simulink library "VariableOrderDifferentialEquationsToolbox"  (R2020a)
settings: Solver=VariableStepAuto  StartTime=0.0  StopTime=10.0  RelTol=1e-3
(part 2 of 3)

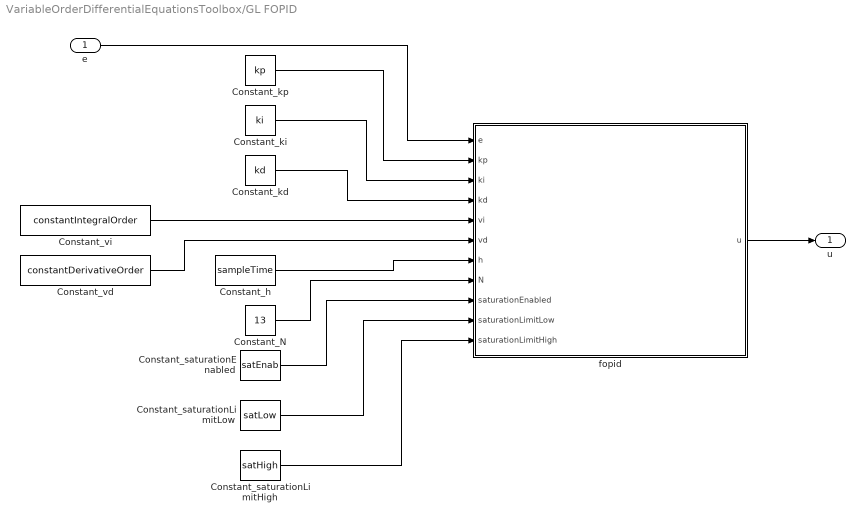
== system VariableOrderDifferentialEquationsToolbox/GL FOPID ==
  e : Inport
  Constant_N : Constant  Value=13
  Constant_h : Constant  Value=sampleTime
  Constant_kd : Constant  Value=kd
  Constant_ki : Constant  Value=ki
  Constant_kp : Constant  Value=kp
  Constant_saturationEnabled : Constant  Value=satEnab
  Constant_saturationLimitHigh : Constant  Value=satHigh
  Constant_saturationLimitLow : Constant  Value=satLow
  Constant_vd : Constant  Value=constantDerivativeOrder
  Constant_vi : Constant  Value=constantIntegralOrder
  fopid : MATLAB Function  TreatAsAtomicUnit=on  SystemSampleTime=1
  u : Outport  VectorParamsAs1DForOutWhenUnconnected=off
  wires:
  Constant_saturationLimitHigh/1 -> fopid/11(saturationLimitHigh)
  e/1 -> fopid/1(e)
  Constant_N/1 -> fopid/8(N)
  Constant_h/1 -> fopid/7(h)
  Constant_kp/1 -> fopid/2(kp)
  Constant_saturationLimitLow/1 -> fopid/10(saturationLimitLow)
  fopid/1(u) -> u/1
  Constant_saturationEnabled/1 -> fopid/9(saturationEnabled)
  Constant_kd/1 -> fopid/4(kd)
  Constant_ki/1 -> fopid/3(ki)
  Constant_vi/1 -> fopid/5(vi)
  Constant_vd/1 -> fopid/6(vd)

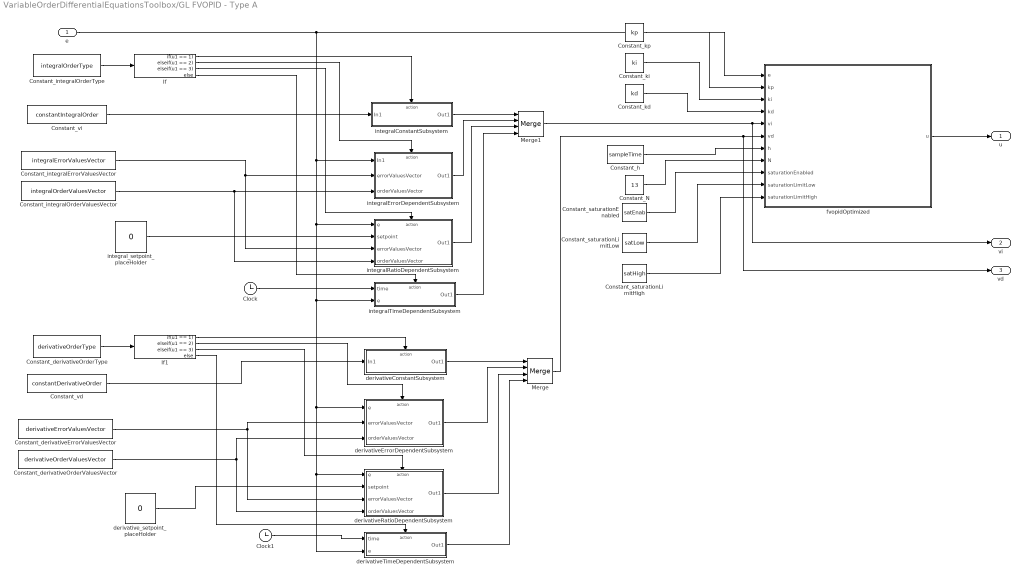
== system VariableOrderDifferentialEquationsToolbox/GL FVOPID - Type A ==
  e : Inport
  Clock : Clock
  Clock1 : Clock
  Constant_N : Constant  Value=13
  Constant_derivativeErrorValuesVector : Constant  Value=derivativeErrorValuesVector
  Constant_derivativeOrderType : Constant  Value=derivativeOrderType
  Constant_derivativeOrderValuesVector : Constant  Value=derivativeOrderValuesVector
  Constant_h : Constant  Value=sampleTime
  Constant_integralErrorValuesVector : Constant  Value=integralErrorValuesVector
  Constant_integralOrderType : Constant  Value=integralOrderType
  Constant_integralOrderValuesVector : Constant  Value=integralOrderValuesVector
  Constant_kd : Constant  Value=kd
  Constant_ki : Constant  Value=ki
  Constant_kp : Constant  Value=kp
  Constant_saturationEnabled : Constant  Value=satEnab
  Constant_saturationLimitHigh : Constant  Value=satHigh
  Constant_saturationLimitLow : Constant  Value=satLow
  Constant_vd : Constant  Value=constantDerivativeOrder
  Constant_vi : Constant  Value=constantIntegralOrder
  If : If  IfExpression=u1 == 1  ElseIfExpressions=u1 == 2, u1 == 3
  If1 : If  IfExpression=u1 == 1  ElseIfExpressions=u1 == 2, u1 == 3
  Merge : Merge  Inputs=4
  Merge1 : Merge  Inputs=4
  derivativeConstantSubsystem : Subsystem  TreatAsAtomicUnit=on
  derivativeErrorDependentSubsystem : Subsystem  TreatAsAtomicUnit=on
  derivativeRatioDependentSubsystem : Subsystem  TreatAsAtomicUnit=on
  derivativeTimeDependentSubsystem : Subsystem  TreatAsAtomicUnit=on
  derivative_setpoint_placeHolder : Constant  Value=0
  fvopidOptimized : MATLAB Function  TreatAsAtomicUnit=on  SystemSampleTime=1
  integralConstantSubsystem : Subsystem  TreatAsAtomicUnit=on
  integralErrorDependentSubsystem : Subsystem  TreatAsAtomicUnit=on
  integralRatioDependentSubsystem : Subsystem  TreatAsAtomicUnit=on
  integralTimeDependentSubsystem : Subsystem  TreatAsAtomicUnit=on
  integral_setpoint_placeHolder : Constant  Value=0
  u : Outport  VectorParamsAs1DForOutWhenUnconnected=off
  vi : Outport  Port=2  VectorParamsAs1DForOutWhenUnconnected=off
  vd : Outport  Port=3  VectorParamsAs1DForOutWhenUnconnected=off
  wires:
  Constant_saturationLimitHigh/1 -> fvopidOptimized/11(saturationLimitHigh)
  e/1 -> fvopidOptimized/1(e), integralErrorDependentSubsystem/1(In1), integralRatioDependentSubsystem/1(e), integralTimeDependentSubsystem/2(e), derivativeTimeDependentSubsystem/2(e), derivativeRatioDependentSubsystem/1(e), derivativeErrorDependentSubsystem/1(e)
  Constant_N/1 -> fvopidOptimized/8(N)
  Constant_h/1 -> fvopidOptimized/7(h)
  Constant_kp/1 -> fvopidOptimized/2(kp)
  Constant_saturationLimitLow/1 -> fvopidOptimized/10(saturationLimitLow)
  fvopidOptimized/1(u) -> u/1
  Constant_saturationEnabled/1 -> fvopidOptimized/9(saturationEnabled)
  Constant_kd/1 -> fvopidOptimized/4(kd)
  Constant_ki/1 -> fvopidOptimized/3(ki)
  Merge1/1 -> vi/1, fvopidOptimized/5(vi)
  Merge/1 -> vd/1, fvopidOptimized/6(vd)
  Constant_integralOrderType/1 -> If/1
  integralConstantSubsystem/1(Out1) -> Merge1/1
  integralErrorDependentSubsystem/1(Out1) -> Merge1/2
  Constant_vi/1 -> integralConstantSubsystem/1(In1)
  If/1 -> integralConstantSubsystem/Action
  Constant_integralErrorValuesVector/1 -> integralErrorDependentSubsystem/2(errorValuesVector), integralRatioDependentSubsystem/3(errorValuesVector)
  Constant_integralOrderValuesVector/1 -> integralRatioDependentSubsystem/4(orderValuesVector), integralErrorDependentSubsystem/3(orderValuesVector)
  integralRatioDependentSubsystem/1(Out1) -> Merge1/3
  If/2 -> integralErrorDependentSubsystem/Action
  If/4 -> integralTimeDependentSubsystem/Action
  Constant_derivativeOrderType/1 -> If1/1
  Constant_vd/1 -> derivativeConstantSubsystem/1(In1)
  derivativeConstantSubsystem/1(Out1) -> Merge/1
  If1/1 -> derivativeConstantSubsystem/Action
  If1/2 -> derivativeErrorDependentSubsystem/Action
  Constant_derivativeErrorValuesVector/1 -> derivativeErrorDependentSubsystem/2(errorValuesVector), derivativeRatioDependentSubsystem/3(errorValuesVector)
  Constant_derivativeOrderValuesVector/1 -> derivativeErrorDependentSubsystem/3(orderValuesVector), derivativeRatioDependentSubsystem/4(orderValuesVector)
  derivativeErrorDependentSubsystem/1(Out1) -> Merge/2
  derivativeRatioDependentSubsystem/1(Out1) -> Merge/3
  Clock/1 -> integralTimeDependentSubsystem/1(time)
  integralTimeDependentSubsystem/1(Out1) -> Merge1/4
  If/3 -> integralRatioDependentSubsystem/Action
  If1/3 -> derivativeRatioDependentSubsystem/Action
  If1/4 -> derivativeTimeDependentSubsystem/Action
  Clock1/1 -> derivativeTimeDependentSubsystem/1(time)
  derivativeTimeDependentSubsystem/1(Out1) -> Merge/4
  integral_setpoint_placeHolder/1 -> integralRatioDependentSubsystem/2(setpoint)
  derivative_setpoint_placeHolder/1 -> derivativeRatioDependentSubsystem/2(setpoint)

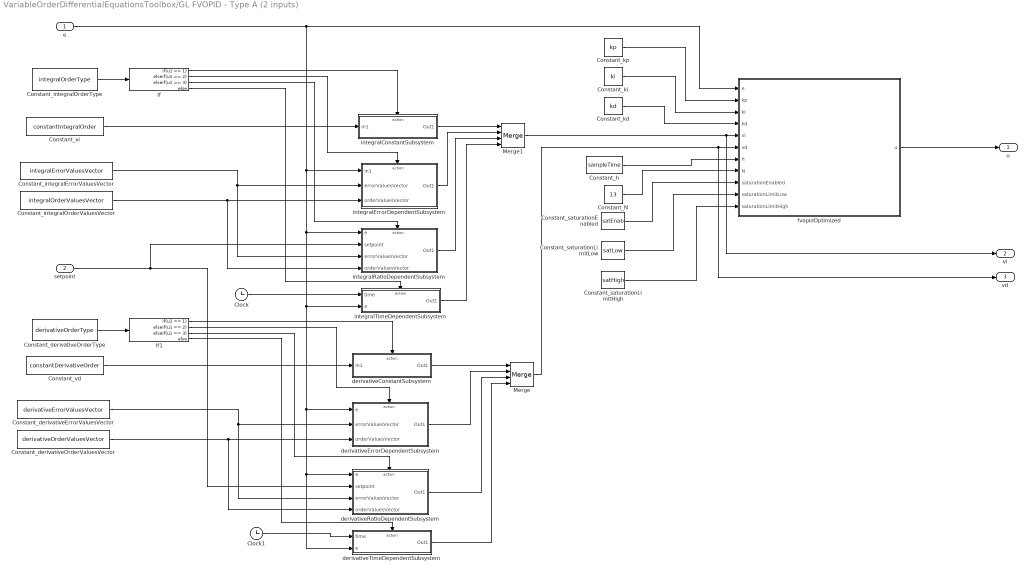
== system VariableOrderDifferentialEquationsToolbox/GL FVOPID - Type A (2 inputs) ==
  e : Inport
  setpoint : Inport  Port=2
  Clock : Clock
  Clock1 : Clock
  Constant_N : Constant  Value=13
  Constant_derivativeErrorValuesVector : Constant  Value=derivativeErrorValuesVector
  Constant_derivativeOrderType : Constant  Value=derivativeOrderType
  Constant_derivativeOrderValuesVector : Constant  Value=derivativeOrderValuesVector
  Constant_h : Constant  Value=sampleTime
  Constant_integralErrorValuesVector : Constant  Value=integralErrorValuesVector
  Constant_integralOrderType : Constant  Value=integralOrderType
  Constant_integralOrderValuesVector : Constant  Value=integralOrderValuesVector
  Constant_kd : Constant  Value=kd
  Constant_ki : Constant  Value=ki
  Constant_kp : Constant  Value=kp
  Constant_saturationEnabled : Constant  Value=satEnab
  Constant_saturationLimitHigh : Constant  Value=satHigh
  Constant_saturationLimitLow : Constant  Value=satLow
  Constant_vd : Constant  Value=constantDerivativeOrder
  Constant_vi : Constant  Value=constantIntegralOrder
  If : If  IfExpression=u1 == 1  ElseIfExpressions=u1 == 2, u1 == 3
  If1 : If  IfExpression=u1 == 1  ElseIfExpressions=u1 == 2, u1 == 3
  Merge : Merge  Inputs=4
  Merge1 : Merge  Inputs=4
  derivativeConstantSubsystem : Subsystem  TreatAsAtomicUnit=on
  derivativeErrorDependentSubsystem : Subsystem  TreatAsAtomicUnit=on
  derivativeRatioDependentSubsystem : Subsystem  TreatAsAtomicUnit=on
  derivativeTimeDependentSubsystem : Subsystem  TreatAsAtomicUnit=on
  fvopidOptimized : MATLAB Function  TreatAsAtomicUnit=on  SystemSampleTime=1
  integralConstantSubsystem : Subsystem  TreatAsAtomicUnit=on
  integralErrorDependentSubsystem : Subsystem  TreatAsAtomicUnit=on
  integralRatioDependentSubsystem : Subsystem  TreatAsAtomicUnit=on
  integralTimeDependentSubsystem : Subsystem  TreatAsAtomicUnit=on
  u : Outport  VectorParamsAs1DForOutWhenUnconnected=off
  vi : Outport  Port=2  VectorParamsAs1DForOutWhenUnconnected=off
  vd : Outport  Port=3  VectorParamsAs1DForOutWhenUnconnected=off
  wires:
  Constant_saturationLimitHigh/1 -> fvopidOptimized/11(saturationLimitHigh)
  e/1 -> integralErrorDependentSubsystem/1(In1), integralRatioDependentSubsystem/1(e), integralTimeDependentSubsystem/2(e), derivativeTimeDependentSubsystem/2(e), derivativeRatioDependentSubsystem/1(e), derivativeErrorDependentSubsystem/1(e), fvopidOptimized/1(e)
  Constant_N/1 -> fvopidOptimized/8(N)
  Constant_h/1 -> fvopidOptimized/7(h)
  Constant_kp/1 -> fvopidOptimized/2(kp)
  Constant_saturationLimitLow/1 -> fvopidOptimized/10(saturationLimitLow)
  fvopidOptimized/1(u) -> u/1
  Constant_saturationEnabled/1 -> fvopidOptimized/9(saturationEnabled)
  Constant_kd/1 -> fvopidOptimized/4(kd)
  Constant_ki/1 -> fvopidOptimized/3(ki)
  Merge1/1 -> vi/1, fvopidOptimized/5(vi)
  Merge/1 -> vd/1, fvopidOptimized/6(vd)
  Constant_integralOrderType/1 -> If/1
  integralConstantSubsystem/1(Out1) -> Merge1/1
  integralErrorDependentSubsystem/1(Out1) -> Merge1/2
  Constant_vi/1 -> integralConstantSubsystem/1(In1)
  If/1 -> integralConstantSubsystem/Action
  Constant_integralErrorValuesVector/1 -> integralErrorDependentSubsystem/2(errorValuesVector), integralRatioDependentSubsystem/3(errorValuesVector)
  Constant_integralOrderValuesVector/1 -> integralRatioDependentSubsystem/4(orderValuesVector), integralErrorDependentSubsystem/3(orderValuesVector)
  integralRatioDependentSubsystem/1(Out1) -> Merge1/3
  If/2 -> integralErrorDependentSubsystem/Action
  If/4 -> integralTimeDependentSubsystem/Action
  Constant_derivativeOrderType/1 -> If1/1
  Constant_vd/1 -> derivativeConstantSubsystem/1(In1)
  derivativeConstantSubsystem/1(Out1) -> Merge/1
  If1/1 -> derivativeConstantSubsystem/Action
  If1/2 -> derivativeErrorDependentSubsystem/Action
  Constant_derivativeErrorValuesVector/1 -> derivativeRatioDependentSubsystem/3(errorValuesVector), derivativeErrorDependentSubsystem/2(errorValuesVector)
  Constant_derivativeOrderValuesVector/1 -> derivativeRatioDependentSubsystem/4(orderValuesVector), derivativeErrorDependentSubsystem/3(orderValuesVector)
  derivativeErrorDependentSubsystem/1(Out1) -> Merge/2
  derivativeRatioDependentSubsystem/1(Out1) -> Merge/3
  Clock/1 -> integralTimeDependentSubsystem/1(time)
  integralTimeDependentSubsystem/1(Out1) -> Merge1/4
  If/3 -> integralRatioDependentSubsystem/Action
  If1/3 -> derivativeRatioDependentSubsystem/Action
  If1/4 -> derivativeTimeDependentSubsystem/Action
  Clock1/1 -> derivativeTimeDependentSubsystem/1(time)
  derivativeTimeDependentSubsystem/1(Out1) -> Merge/4
  setpoint/1 -> integralRatioDependentSubsystem/2(setpoint), derivativeRatioDependentSubsystem/2(setpoint)

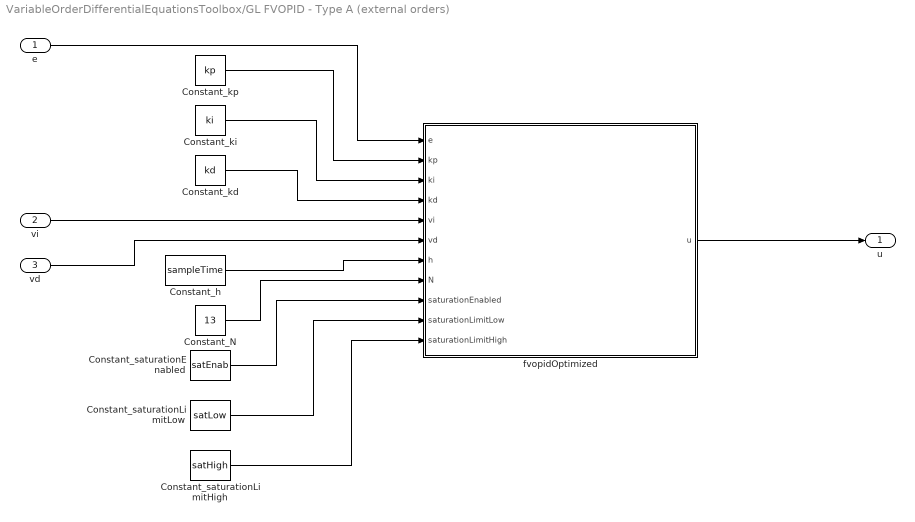
== system VariableOrderDifferentialEquationsToolbox/GL FVOPID - Type A (external orders) ==
  e : Inport
  vi : Inport  Port=2
  vd : Inport  Port=3
  Constant_N : Constant  Value=13
  Constant_h : Constant  Value=sampleTime
  Constant_kd : Constant  Value=kd
  Constant_ki : Constant  Value=ki
  Constant_kp : Constant  Value=kp
  Constant_saturationEnabled : Constant  Value=satEnab
  Constant_saturationLimitHigh : Constant  Value=satHigh
  Constant_saturationLimitLow : Constant  Value=satLow
  fvopidOptimized : MATLAB Function  TreatAsAtomicUnit=on  SystemSampleTime=1
  u : Outport  VectorParamsAs1DForOutWhenUnconnected=off
  wires:
  Constant_saturationLimitHigh/1 -> fvopidOptimized/11(saturationLimitHigh)
  e/1 -> fvopidOptimized/1(e)
  Constant_N/1 -> fvopidOptimized/8(N)
  Constant_h/1 -> fvopidOptimized/7(h)
  Constant_kp/1 -> fvopidOptimized/2(kp)
  Constant_saturationLimitLow/1 -> fvopidOptimized/10(saturationLimitLow)
  fvopidOptimized/1(u) -> u/1
  Constant_saturationEnabled/1 -> fvopidOptimized/9(saturationEnabled)
  Constant_kd/1 -> fvopidOptimized/4(kd)
  Constant_ki/1 -> fvopidOptimized/3(ki)
  vi/1 -> fvopidOptimized/5(vi)
  vd/1 -> fvopidOptimized/6(vd)

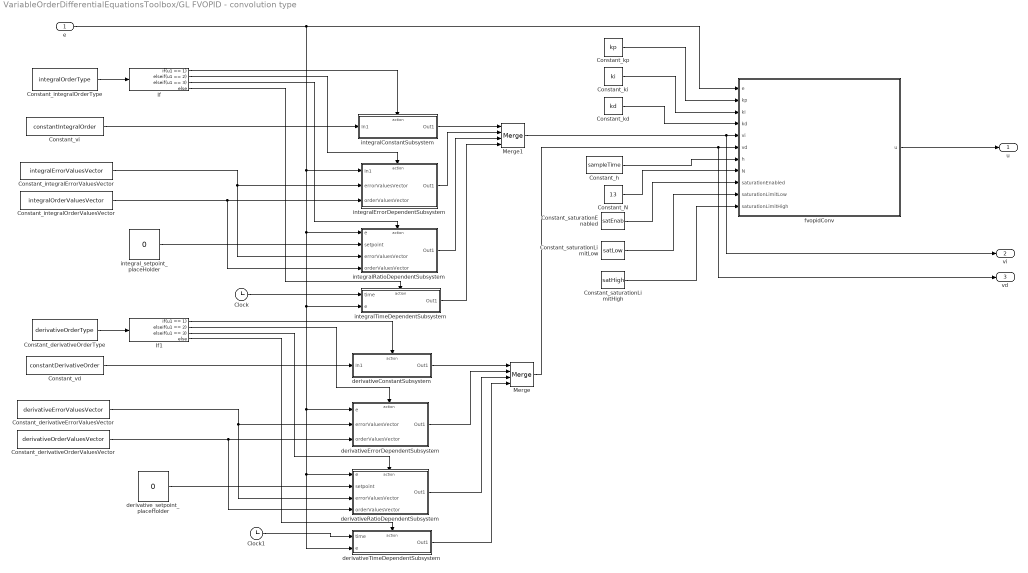
== system VariableOrderDifferentialEquationsToolbox/GL FVOPID - convolution type ==
  e : Inport
  Clock : Clock
  Clock1 : Clock
  Constant_N : Constant  Value=13
  Constant_derivativeErrorValuesVector : Constant  Value=derivativeErrorValuesVector
  Constant_derivativeOrderType : Constant  Value=derivativeOrderType
  Constant_derivativeOrderValuesVector : Constant  Value=derivativeOrderValuesVector
  Constant_h : Constant  Value=sampleTime
  Constant_integralErrorValuesVector : Constant  Value=integralErrorValuesVector
  Constant_integralOrderType : Constant  Value=integralOrderType
  Constant_integralOrderValuesVector : Constant  Value=integralOrderValuesVector
  Constant_kd : Constant  Value=kd
  Constant_ki : Constant  Value=ki
  Constant_kp : Constant  Value=kp
  Constant_saturationEnabled : Constant  Value=satEnab
  Constant_saturationLimitHigh : Constant  Value=satHigh
  Constant_saturationLimitLow : Constant  Value=satLow
  Constant_vd : Constant  Value=constantDerivativeOrder
  Constant_vi : Constant  Value=constantIntegralOrder
  If : If  IfExpression=u1 == 1  ElseIfExpressions=u1 == 2, u1 == 3
  If1 : If  IfExpression=u1 == 1  ElseIfExpressions=u1 == 2, u1 == 3
  Merge : Merge  Inputs=4
  Merge1 : Merge  Inputs=4
  derivativeConstantSubsystem : Subsystem  TreatAsAtomicUnit=on
  derivativeErrorDependentSubsystem : Subsystem  TreatAsAtomicUnit=on
  derivativeRatioDependentSubsystem : Subsystem  TreatAsAtomicUnit=on
  derivativeTimeDependentSubsystem : Subsystem  TreatAsAtomicUnit=on
  derivative_setpoint_placeHolder : Constant  Value=0
  fvopidConv : MATLAB Function  TreatAsAtomicUnit=on  SystemSampleTime=1
  integralConstantSubsystem : Subsystem  TreatAsAtomicUnit=on
  integralErrorDependentSubsystem : Subsystem  TreatAsAtomicUnit=on
  integralRatioDependentSubsystem : Subsystem  TreatAsAtomicUnit=on
  integralTimeDependentSubsystem : Subsystem  TreatAsAtomicUnit=on
  integral_setpoint_placeHolder : Constant  Value=0
  u : Outport  VectorParamsAs1DForOutWhenUnconnected=off
  vi : Outport  Port=2  VectorParamsAs1DForOutWhenUnconnected=off
  vd : Outport  Port=3  VectorParamsAs1DForOutWhenUnconnected=off
  wires:
  Constant_saturationLimitHigh/1 -> fvopidConv/11(saturationLimitHigh)
  e/1 -> integralErrorDependentSubsystem/1(In1), integralRatioDependentSubsystem/1(e), integralTimeDependentSubsystem/2(e), derivativeTimeDependentSubsystem/2(e), derivativeRatioDependentSubsystem/1(e), derivativeErrorDependentSubsystem/1(e), fvopidConv/1(e)
  Constant_N/1 -> fvopidConv/8(N)
  Constant_h/1 -> fvopidConv/7(h)
  Constant_kp/1 -> fvopidConv/2(kp)
  Constant_saturationLimitLow/1 -> fvopidConv/10(saturationLimitLow)
  fvopidConv/1(u) -> u/1
  Constant_saturationEnabled/1 -> fvopidConv/9(saturationEnabled)
  Constant_kd/1 -> fvopidConv/4(kd)
  Constant_ki/1 -> fvopidConv/3(ki)
  Merge1/1 -> vi/1, fvopidConv/5(vi)
  Merge/1 -> vd/1, fvopidConv/6(vd)
  Constant_integralOrderType/1 -> If/1
  integralConstantSubsystem/1(Out1) -> Merge1/1
  integralErrorDependentSubsystem/1(Out1) -> Merge1/2
  Constant_vi/1 -> integralConstantSubsystem/1(In1)
  If/1 -> integralConstantSubsystem/Action
  Constant_integralErrorValuesVector/1 -> integralErrorDependentSubsystem/2(errorValuesVector), integralRatioDependentSubsystem/3(errorValuesVector)
  Constant_integralOrderValuesVector/1 -> integralRatioDependentSubsystem/4(orderValuesVector), integralErrorDependentSubsystem/3(orderValuesVector)
  integralRatioDependentSubsystem/1(Out1) -> Merge1/3
  If/2 -> integralErrorDependentSubsystem/Action
  If/4 -> integralTimeDependentSubsystem/Action
  Constant_derivativeOrderType/1 -> If1/1
  Constant_vd/1 -> derivativeConstantSubsystem/1(In1)
  derivativeConstantSubsystem/1(Out1) -> Merge/1
  If1/1 -> derivativeConstantSubsystem/Action
  If1/2 -> derivativeErrorDependentSubsystem/Action
  Constant_derivativeErrorValuesVector/1 -> derivativeRatioDependentSubsystem/3(errorValuesVector), derivativeErrorDependentSubsystem/2(errorValuesVector)
  Constant_derivativeOrderValuesVector/1 -> derivativeRatioDependentSubsystem/4(orderValuesVector), derivativeErrorDependentSubsystem/3(orderValuesVector)
  derivativeErrorDependentSubsystem/1(Out1) -> Merge/2
  derivativeRatioDependentSubsystem/1(Out1) -> Merge/3
  Clock/1 -> integralTimeDependentSubsystem/1(time)
  integralTimeDependentSubsystem/1(Out1) -> Merge1/4
  If/3 -> integralRatioDependentSubsystem/Action
  If1/3 -> derivativeRatioDependentSubsystem/Action
  If1/4 -> derivativeTimeDependentSubsystem/Action
  Clock1/1 -> derivativeTimeDependentSubsystem/1(time)
  derivativeTimeDependentSubsystem/1(Out1) -> Merge/4
  integral_setpoint_placeHolder/1 -> integralRatioDependentSubsystem/2(setpoint)
  derivative_setpoint_placeHolder/1 -> derivativeRatioDependentSubsystem/2(setpoint)

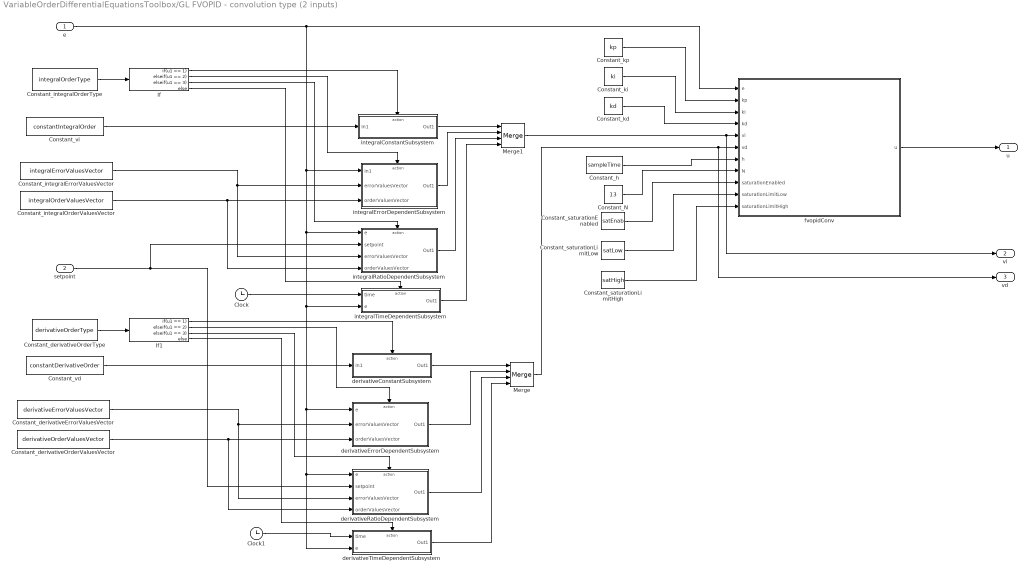
== system VariableOrderDifferentialEquationsToolbox/GL FVOPID - convolution type (2 inputs) ==
  e : Inport
  setpoint : Inport  Port=2
  Clock : Clock
  Clock1 : Clock
  Constant_N : Constant  Value=13
  Constant_derivativeErrorValuesVector : Constant  Value=derivativeErrorValuesVector
  Constant_derivativeOrderType : Constant  Value=derivativeOrderType
  Constant_derivativeOrderValuesVector : Constant  Value=derivativeOrderValuesVector
  Constant_h : Constant  Value=sampleTime
  Constant_integralErrorValuesVector : Constant  Value=integralErrorValuesVector
  Constant_integralOrderType : Constant  Value=integralOrderType
  Constant_integralOrderValuesVector : Constant  Value=integralOrderValuesVector
  Constant_kd : Constant  Value=kd
  Constant_ki : Constant  Value=ki
  Constant_kp : Constant  Value=kp
  Constant_saturationEnabled : Constant  Value=satEnab
  Constant_saturationLimitHigh : Constant  Value=satHigh
  Constant_saturationLimitLow : Constant  Value=satLow
  Constant_vd : Constant  Value=constantDerivativeOrder
  Constant_vi : Constant  Value=constantIntegralOrder
  If : If  IfExpression=u1 == 1  ElseIfExpressions=u1 == 2, u1 == 3
  If1 : If  IfExpression=u1 == 1  ElseIfExpressions=u1 == 2, u1 == 3
  Merge : Merge  Inputs=4
  Merge1 : Merge  Inputs=4
  derivativeConstantSubsystem : Subsystem  TreatAsAtomicUnit=on
  derivativeErrorDependentSubsystem : Subsystem  TreatAsAtomicUnit=on
  derivativeRatioDependentSubsystem : Subsystem  TreatAsAtomicUnit=on
  derivativeTimeDependentSubsystem : Subsystem  TreatAsAtomicUnit=on
  fvopidConv : MATLAB Function  TreatAsAtomicUnit=on  SystemSampleTime=1
  integralConstantSubsystem : Subsystem  TreatAsAtomicUnit=on
  integralErrorDependentSubsystem : Subsystem  TreatAsAtomicUnit=on
  integralRatioDependentSubsystem : Subsystem  TreatAsAtomicUnit=on
  integralTimeDependentSubsystem : Subsystem  TreatAsAtomicUnit=on
  u : Outport  VectorParamsAs1DForOutWhenUnconnected=off
  vi : Outport  Port=2  VectorParamsAs1DForOutWhenUnconnected=off
  vd : Outport  Port=3  VectorParamsAs1DForOutWhenUnconnected=off
  wires:
  Constant_saturationLimitHigh/1 -> fvopidConv/11(saturationLimitHigh)
  e/1 -> integralErrorDependentSubsystem/1(In1), integralRatioDependentSubsystem/1(e), integralTimeDependentSubsystem/2(e), derivativeTimeDependentSubsystem/2(e), derivativeRatioDependentSubsystem/1(e), derivativeErrorDependentSubsystem/1(e), fvopidConv/1(e)
  Constant_N/1 -> fvopidConv/8(N)
  Constant_h/1 -> fvopidConv/7(h)
  Constant_kp/1 -> fvopidConv/2(kp)
  Constant_saturationLimitLow/1 -> fvopidConv/10(saturationLimitLow)
  fvopidConv/1(u) -> u/1
  Constant_saturationEnabled/1 -> fvopidConv/9(saturationEnabled)
  Constant_kd/1 -> fvopidConv/4(kd)
  Constant_ki/1 -> fvopidConv/3(ki)
  Merge1/1 -> vi/1, fvopidConv/5(vi)
  Merge/1 -> vd/1, fvopidConv/6(vd)
  Constant_integralOrderType/1 -> If/1
  integralConstantSubsystem/1(Out1) -> Merge1/1
  integralErrorDependentSubsystem/1(Out1) -> Merge1/2
  Constant_vi/1 -> integralConstantSubsystem/1(In1)
  If/1 -> integralConstantSubsystem/Action
  Constant_integralErrorValuesVector/1 -> integralErrorDependentSubsystem/2(errorValuesVector), integralRatioDependentSubsystem/3(errorValuesVector)
  Constant_integralOrderValuesVector/1 -> integralRatioDependentSubsystem/4(orderValuesVector), integralErrorDependentSubsystem/3(orderValuesVector)
  integralRatioDependentSubsystem/1(Out1) -> Merge1/3
  If/2 -> integralErrorDependentSubsystem/Action
  If/4 -> integralTimeDependentSubsystem/Action
  Constant_derivativeOrderType/1 -> If1/1
  Constant_vd/1 -> derivativeConstantSubsystem/1(In1)
  derivativeConstantSubsystem/1(Out1) -> Merge/1
  If1/1 -> derivativeConstantSubsystem/Action
  If1/2 -> derivativeErrorDependentSubsystem/Action
  Constant_derivativeErrorValuesVector/1 -> derivativeRatioDependentSubsystem/3(errorValuesVector), derivativeErrorDependentSubsystem/2(errorValuesVector)
  Constant_derivativeOrderValuesVector/1 -> derivativeRatioDependentSubsystem/4(orderValuesVector), derivativeErrorDependentSubsystem/3(orderValuesVector)
  derivativeErrorDependentSubsystem/1(Out1) -> Merge/2
  derivativeRatioDependentSubsystem/1(Out1) -> Merge/3
  Clock/1 -> integralTimeDependentSubsystem/1(time)
  integralTimeDependentSubsystem/1(Out1) -> Merge1/4
  If/3 -> integralRatioDependentSubsystem/Action
  If1/3 -> derivativeRatioDependentSubsystem/Action
  If1/4 -> derivativeTimeDependentSubsystem/Action
  Clock1/1 -> derivativeTimeDependentSubsystem/1(time)
  derivativeTimeDependentSubsystem/1(Out1) -> Merge/4
  setpoint/1 -> integralRatioDependentSubsystem/2(setpoint), derivativeRatioDependentSubsystem/2(setpoint)

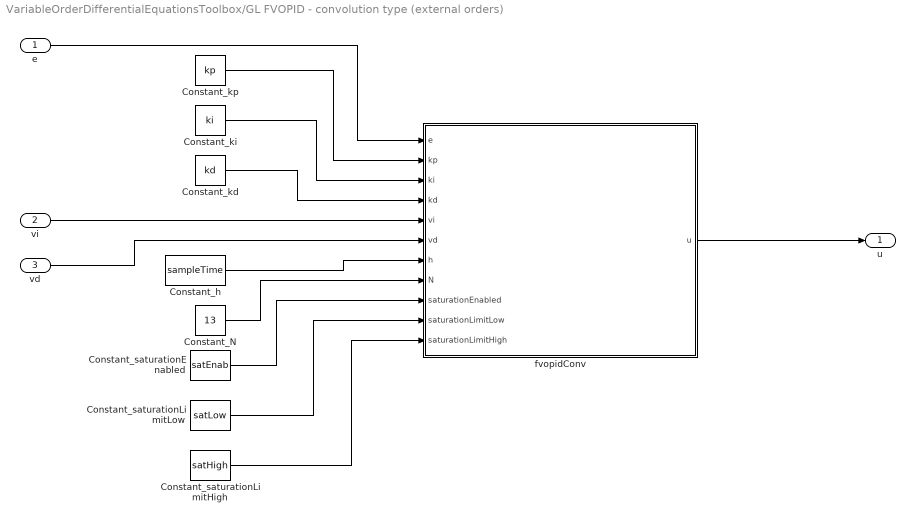
== system VariableOrderDifferentialEquationsToolbox/GL FVOPID - convolution type (external orders) ==
  e : Inport
  vi : Inport  Port=2
  vd : Inport  Port=3
  Constant_N : Constant  Value=13
  Constant_h : Constant  Value=sampleTime
  Constant_kd : Constant  Value=kd
  Constant_ki : Constant  Value=ki
  Constant_kp : Constant  Value=kp
  Constant_saturationEnabled : Constant  Value=satEnab
  Constant_saturationLimitHigh : Constant  Value=satHigh
  Constant_saturationLimitLow : Constant  Value=satLow
  fvopidConv : MATLAB Function  TreatAsAtomicUnit=on  SystemSampleTime=1
  u : Outport  VectorParamsAs1DForOutWhenUnconnected=off
  wires:
  Constant_saturationLimitHigh/1 -> fvopidConv/11(saturationLimitHigh)
  e/1 -> fvopidConv/1(e)
  Constant_N/1 -> fvopidConv/8(N)
  Constant_h/1 -> fvopidConv/7(h)
  Constant_kp/1 -> fvopidConv/2(kp)
  Constant_saturationLimitLow/1 -> fvopidConv/10(saturationLimitLow)
  fvopidConv/1(u) -> u/1
  Constant_saturationEnabled/1 -> fvopidConv/9(saturationEnabled)
  Constant_kd/1 -> fvopidConv/4(kd)
  Constant_ki/1 -> fvopidConv/3(ki)
  vi/1 -> fvopidConv/5(vi)
  vd/1 -> fvopidConv/6(vd)

== system VariableOrderDifferentialEquationsToolbox/GL FVOPID - Type A/derivativeConstantSubsystem ==
  In1 : Inport
  Action Port : ActionPort  ActionPortLabel=if { }
  Out1 : Outport  VectorParamsAs1DForOutWhenUnconnected=off
  wires:
  In1/1 -> Out1/1

== system VariableOrderDifferentialEquationsToolbox/GL FVOPID - Type A/derivativeErrorDependentSubsystem ==
  e : Inport
  errorValuesVector : Inport  Port=2
  orderValuesVector : Inport  Port=3
  Action Port : ActionPort  ActionPortLabel=elseif { }
  Derivative Error Depenent Order : MATLAB Function  TreatAsAtomicUnit=on
  Out1 : Outport  VectorParamsAs1DForOutWhenUnconnected=off
  wires:
  e/1 -> Derivative Error Depenent Order/1(e)
  Derivative Error Depenent Order/1(y) -> Out1/1
  errorValuesVector/1 -> Derivative Error Depenent Order/2(errorValuesVector)
  orderValuesVector/1 -> Derivative Error Depenent Order/3(orderValuesVector)

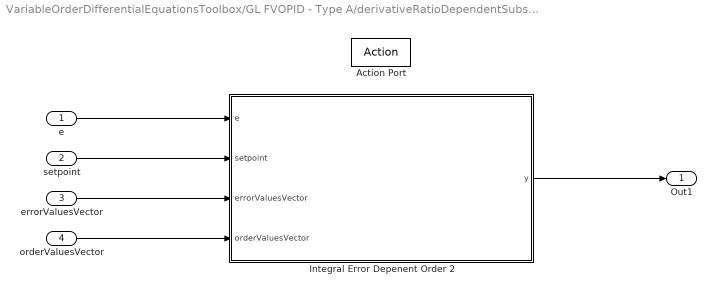
== system VariableOrderDifferentialEquationsToolbox/GL FVOPID - Type A/derivativeRatioDependentSubsystem ==
  e : Inport
  setpoint : Inport  Port=2
  errorValuesVector : Inport  Port=3
  orderValuesVector : Inport  Port=4
  Action Port : ActionPort  ActionPortLabel=elseif { }
  Integral Error Depenent Order 2 : MATLAB Function  TreatAsAtomicUnit=on
  Out1 : Outport  VectorParamsAs1DForOutWhenUnconnected=off
  wires:
  e/1 -> Integral Error Depenent Order 2/1(e)
  Integral Error Depenent Order 2/1(y) -> Out1/1
  errorValuesVector/1 -> Integral Error Depenent Order 2/3(errorValuesVector)
  orderValuesVector/1 -> Integral Error Depenent Order 2/4(orderValuesVector)
  setpoint/1 -> Integral Error Depenent Order 2/2(setpoint)

== system VariableOrderDifferentialEquationsToolbox/GL FVOPID - Type A/derivativeTimeDependentSubsystem ==
  time : Inport
  e : Inport  Port=2
  Action Port : ActionPort  ActionPortLabel=else { }
  derivativeTimeDependentBlock : MATLAB Function  TreatAsAtomicUnit=on
  Out1 : Outport  VectorParamsAs1DForOutWhenUnconnected=off
  wires:
  time/1 -> derivativeTimeDependentBlock/1(t)
  derivativeTimeDependentBlock/1(y) -> Out1/1
  e/1 -> derivativeTimeDependentBlock/2(e)

== system VariableOrderDifferentialEquationsToolbox/GL FVOPID - Type A/integralConstantSubsystem ==
  In1 : Inport
  Action Port : ActionPort  ActionPortLabel=if { }
  Out1 : Outport  VectorParamsAs1DForOutWhenUnconnected=off
  wires:
  In1/1 -> Out1/1

== system VariableOrderDifferentialEquationsToolbox/GL FVOPID - Type A/integralErrorDependentSubsystem ==
  In1 : Inport
  errorValuesVector : Inport  Port=2
  orderValuesVector : Inport  Port=3
  Action Port : ActionPort  ActionPortLabel=elseif { }
  Integral Error Depenent Order : MATLAB Function  TreatAsAtomicUnit=on
  Out1 : Outport  VectorParamsAs1DForOutWhenUnconnected=off
  wires:
  In1/1 -> Integral Error Depenent Order/1(e)
  Integral Error Depenent Order/1(y) -> Out1/1
  errorValuesVector/1 -> Integral Error Depenent Order/2(errorValuesVector)
  orderValuesVector/1 -> Integral Error Depenent Order/3(orderValuesVector)

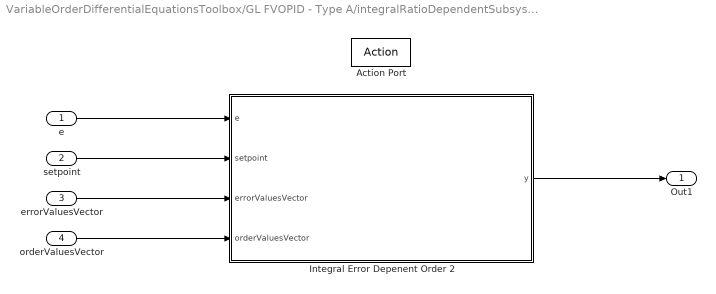
== system VariableOrderDifferentialEquationsToolbox/GL FVOPID - Type A/integralRatioDependentSubsystem ==
  e : Inport
  setpoint : Inport  Port=2
  errorValuesVector : Inport  Port=3
  orderValuesVector : Inport  Port=4
  Action Port : ActionPort  ActionPortLabel=elseif { }
  Integral Error Depenent Order 2 : MATLAB Function  TreatAsAtomicUnit=on
  Out1 : Outport  VectorParamsAs1DForOutWhenUnconnected=off
  wires:
  e/1 -> Integral Error Depenent Order 2/1(e)
  Integral Error Depenent Order 2/1(y) -> Out1/1
  errorValuesVector/1 -> Integral Error Depenent Order 2/3(errorValuesVector)
  orderValuesVector/1 -> Integral Error Depenent Order 2/4(orderValuesVector)
  setpoint/1 -> Integral Error Depenent Order 2/2(setpoint)

== system VariableOrderDifferentialEquationsToolbox/GL FVOPID - Type A/integralTimeDependentSubsystem ==
  time : Inport
  e : Inport  Port=2
  Action Port : ActionPort  ActionPortLabel=else { }
  integralTimeDependentBlock : MATLAB Function  TreatAsAtomicUnit=on
  Out1 : Outport  VectorParamsAs1DForOutWhenUnconnected=off
  wires:
  time/1 -> integralTimeDependentBlock/1(t)
  integralTimeDependentBlock/1(y) -> Out1/1
  e/1 -> integralTimeDependentBlock/2(e)

== system VariableOrderDifferentialEquationsToolbox/GL FVOPID - Type A (2 inputs)/derivativeConstantSubsystem ==
  In1 : Inport
  Action Port : ActionPort
  Out1 : Outport  VectorParamsAs1DForOutWhenUnconnected=off
  wires:
  In1/1 -> Out1/1

== system VariableOrderDifferentialEquationsToolbox/GL FVOPID - Type A (2 inputs)/derivativeErrorDependentSubsystem ==
  e : Inport
  errorValuesVector : Inport  Port=2
  orderValuesVector : Inport  Port=3
  Action Port : ActionPort
  Derivative Error Depenent Order : MATLAB Function  TreatAsAtomicUnit=on
  Out1 : Outport  VectorParamsAs1DForOutWhenUnconnected=off
  wires:
  e/1 -> Derivative Error Depenent Order/1(e)
  Derivative Error Depenent Order/1(y) -> Out1/1
  errorValuesVector/1 -> Derivative Error Depenent Order/2(errorValuesVector)
  orderValuesVector/1 -> Derivative Error Depenent Order/3(orderValuesVector)

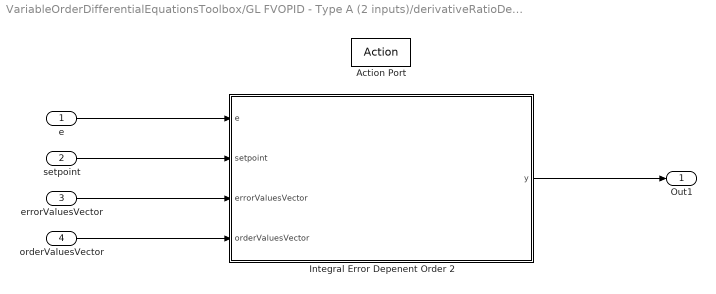
== system VariableOrderDifferentialEquationsToolbox/GL FVOPID - Type A (2 inputs)/derivativeRatioDependentSubsystem ==
  e : Inport
  setpoint : Inport  Port=2
  errorValuesVector : Inport  Port=3
  orderValuesVector : Inport  Port=4
  Action Port : ActionPort
  Integral Error Depenent Order 2 : MATLAB Function  TreatAsAtomicUnit=on
  Out1 : Outport  VectorParamsAs1DForOutWhenUnconnected=off
  wires:
  e/1 -> Integral Error Depenent Order 2/1(e)
  Integral Error Depenent Order 2/1(y) -> Out1/1
  errorValuesVector/1 -> Integral Error Depenent Order 2/3(errorValuesVector)
  orderValuesVector/1 -> Integral Error Depenent Order 2/4(orderValuesVector)
  setpoint/1 -> Integral Error Depenent Order 2/2(setpoint)

== system VariableOrderDifferentialEquationsToolbox/GL FVOPID - Type A (2 inputs)/derivativeTimeDependentSubsystem ==
  time : Inport
  e : Inport  Port=2
  Action Port : ActionPort
  derivativeTimeDependentBlock : MATLAB Function  TreatAsAtomicUnit=on
  Out1 : Outport  VectorParamsAs1DForOutWhenUnconnected=off
  wires:
  time/1 -> derivativeTimeDependentBlock/1(t)
  derivativeTimeDependentBlock/1(y) -> Out1/1
  e/1 -> derivativeTimeDependentBlock/2(e)

== system VariableOrderDifferentialEquationsToolbox/GL FVOPID - Type A (2 inputs)/integralConstantSubsystem ==
  In1 : Inport
  Action Port : ActionPort
  Out1 : Outport  VectorParamsAs1DForOutWhenUnconnected=off
  wires:
  In1/1 -> Out1/1

== system VariableOrderDifferentialEquationsToolbox/GL FVOPID - Type A (2 inputs)/integralErrorDependentSubsystem ==
  In1 : Inport
  errorValuesVector : Inport  Port=2
  orderValuesVector : Inport  Port=3
  Action Port : ActionPort
  Integral Error Depenent Order : MATLAB Function  TreatAsAtomicUnit=on
  Out1 : Outport  VectorParamsAs1DForOutWhenUnconnected=off
  wires:
  In1/1 -> Integral Error Depenent Order/1(e)
  Integral Error Depenent Order/1(y) -> Out1/1
  errorValuesVector/1 -> Integral Error Depenent Order/2(errorValuesVector)
  orderValuesVector/1 -> Integral Error Depenent Order/3(orderValuesVector)

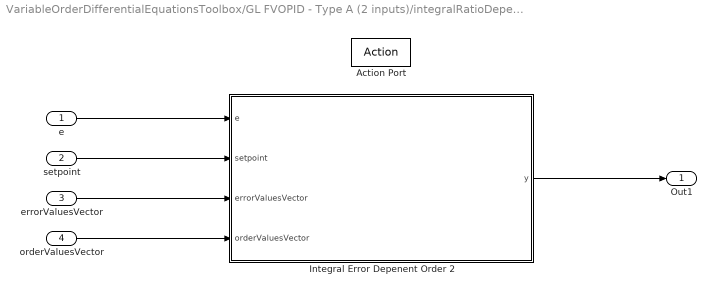
== system VariableOrderDifferentialEquationsToolbox/GL FVOPID - Type A (2 inputs)/integralRatioDependentSubsystem ==
  e : Inport
  setpoint : Inport  Port=2
  errorValuesVector : Inport  Port=3
  orderValuesVector : Inport  Port=4
  Action Port : ActionPort
  Integral Error Depenent Order 2 : MATLAB Function  TreatAsAtomicUnit=on
  Out1 : Outport  VectorParamsAs1DForOutWhenUnconnected=off
  wires:
  e/1 -> Integral Error Depenent Order 2/1(e)
  Integral Error Depenent Order 2/1(y) -> Out1/1
  errorValuesVector/1 -> Integral Error Depenent Order 2/3(errorValuesVector)
  orderValuesVector/1 -> Integral Error Depenent Order 2/4(orderValuesVector)
  setpoint/1 -> Integral Error Depenent Order 2/2(setpoint)

== system VariableOrderDifferentialEquationsToolbox/GL FVOPID - Type A (2 inputs)/integralTimeDependentSubsystem ==
  time : Inport
  e : Inport  Port=2
  Action Port : ActionPort
  integralTimeDependentBlock : MATLAB Function  TreatAsAtomicUnit=on
  Out1 : Outport  VectorParamsAs1DForOutWhenUnconnected=off
  wires:
  time/1 -> integralTimeDependentBlock/1(t)
  integralTimeDependentBlock/1(y) -> Out1/1
  e/1 -> integralTimeDependentBlock/2(e)

== system VariableOrderDifferentialEquationsToolbox/GL FVOPID - convolution type/derivativeConstantSubsystem ==
  In1 : Inport
  Action Port : ActionPort
  Out1 : Outport  VectorParamsAs1DForOutWhenUnconnected=off
  wires:
  In1/1 -> Out1/1

== system VariableOrderDifferentialEquationsToolbox/GL FVOPID - convolution type/derivativeErrorDependentSubsystem ==
  e : Inport
  errorValuesVector : Inport  Port=2
  orderValuesVector : Inport  Port=3
  Action Port : ActionPort
  Derivative Error Depenent Order : MATLAB Function  TreatAsAtomicUnit=on
  Out1 : Outport  VectorParamsAs1DForOutWhenUnconnected=off
  wires:
  e/1 -> Derivative Error Depenent Order/1(e)
  Derivative Error Depenent Order/1(y) -> Out1/1
  errorValuesVector/1 -> Derivative Error Depenent Order/2(errorValuesVector)
  orderValuesVector/1 -> Derivative Error Depenent Order/3(orderValuesVector)

== system VariableOrderDifferentialEquationsToolbox/GL FVOPID - convolution type/derivativeRatioDependentSubsystem ==
  e : Inport
  setpoint : Inport  Port=2
  errorValuesVector : Inport  Port=3
  orderValuesVector : Inport  Port=4
  Action Port : ActionPort
  Integral Error Depenent Order 2 : MATLAB Function  TreatAsAtomicUnit=on
  Out1 : Outport  VectorParamsAs1DForOutWhenUnconnected=off
  wires:
  e/1 -> Integral Error Depenent Order 2/1(e)
  Integral Error Depenent Order 2/1(y) -> Out1/1
  errorValuesVector/1 -> Integral Error Depenent Order 2/3(errorValuesVector)
  orderValuesVector/1 -> Integral Error Depenent Order 2/4(orderValuesVector)
  setpoint/1 -> Integral Error Depenent Order 2/2(setpoint)

== system VariableOrderDifferentialEquationsToolbox/GL FVOPID - convolution type/derivativeTimeDependentSubsystem ==
  time : Inport
  e : Inport  Port=2
  Action Port : ActionPort
  derivativeTimeDependentBlock : MATLAB Function  TreatAsAtomicUnit=on
  Out1 : Outport  VectorParamsAs1DForOutWhenUnconnected=off
  wires:
  time/1 -> derivativeTimeDependentBlock/1(t)
  derivativeTimeDependentBlock/1(y) -> Out1/1
  e/1 -> derivativeTimeDependentBlock/2(e)

== system VariableOrderDifferentialEquationsToolbox/GL FVOPID - convolution type/integralConstantSubsystem ==
  In1 : Inport
  Action Port : ActionPort
  Out1 : Outport  VectorParamsAs1DForOutWhenUnconnected=off
  wires:
  In1/1 -> Out1/1

== system VariableOrderDifferentialEquationsToolbox/GL FVOPID - convolution type/integralErrorDependentSubsystem ==
  In1 : Inport
  errorValuesVector : Inport  Port=2
  orderValuesVector : Inport  Port=3
  Action Port : ActionPort
  Integral Error Depenent Order : MATLAB Function  TreatAsAtomicUnit=on
  Out1 : Outport  VectorParamsAs1DForOutWhenUnconnected=off
  wires:
  In1/1 -> Integral Error Depenent Order/1(e)
  Integral Error Depenent Order/1(y) -> Out1/1
  errorValuesVector/1 -> Integral Error Depenent Order/2(errorValuesVector)
  orderValuesVector/1 -> Integral Error Depenent Order/3(orderValuesVector)

== system VariableOrderDifferentialEquationsToolbox/GL FVOPID - convolution type/integralRatioDependentSubsystem ==
  e : Inport
  setpoint : Inport  Port=2
  errorValuesVector : Inport  Port=3
  orderValuesVector : Inport  Port=4
  Action Port : ActionPort
  Integral Error Depenent Order 2 : MATLAB Function  TreatAsAtomicUnit=on
  Out1 : Outport  VectorParamsAs1DForOutWhenUnconnected=off
  wires:
  e/1 -> Integral Error Depenent Order 2/1(e)
  Integral Error Depenent Order 2/1(y) -> Out1/1
  errorValuesVector/1 -> Integral Error Depenent Order 2/3(errorValuesVector)
  orderValuesVector/1 -> Integral Error Depenent Order 2/4(orderValuesVector)
  setpoint/1 -> Integral Error Depenent Order 2/2(setpoint)

== system VariableOrderDifferentialEquationsToolbox/GL FVOPID - convolution type/integralTimeDependentSubsystem ==
  time : Inport
  e : Inport  Port=2
  Action Port : ActionPort
  integralTimeDependentBlock : MATLAB Function  TreatAsAtomicUnit=on
  Out1 : Outport  VectorParamsAs1DForOutWhenUnconnected=off
  wires:
  time/1 -> integralTimeDependentBlock/1(t)
  integralTimeDependentBlock/1(y) -> Out1/1
  e/1 -> integralTimeDependentBlock/2(e)

== system VariableOrderDifferentialEquationsToolbox/GL FVOPID - convolution type (2 inputs)/derivativeConstantSubsystem ==
  In1 : Inport
  Action Port : ActionPort
  Out1 : Outport  VectorParamsAs1DForOutWhenUnconnected=off
  wires:
  In1/1 -> Out1/1

== system VariableOrderDifferentialEquationsToolbox/GL FVOPID - convolution type (2 inputs)/derivativeErrorDependentSubsystem ==
  e : Inport
  errorValuesVector : Inport  Port=2
  orderValuesVector : Inport  Port=3
  Action Port : ActionPort
  Derivative Error Depenent Order : MATLAB Function  TreatAsAtomicUnit=on
  Out1 : Outport  VectorParamsAs1DForOutWhenUnconnected=off
  wires:
  e/1 -> Derivative Error Depenent Order/1(e)
  Derivative Error Depenent Order/1(y) -> Out1/1
  errorValuesVector/1 -> Derivative Error Depenent Order/2(errorValuesVector)
  orderValuesVector/1 -> Derivative Error Depenent Order/3(orderValuesVector)

== system VariableOrderDifferentialEquationsToolbox/GL FVOPID - convolution type (2 inputs)/derivativeRatioDependentSubsystem ==
  e : Inport
  setpoint : Inport  Port=2
  errorValuesVector : Inport  Port=3
  orderValuesVector : Inport  Port=4
  Action Port : ActionPort
  Integral Error Depenent Order 2 : MATLAB Function  TreatAsAtomicUnit=on
  Out1 : Outport  VectorParamsAs1DForOutWhenUnconnected=off
  wires:
  e/1 -> Integral Error Depenent Order 2/1(e)
  Integral Error Depenent Order 2/1(y) -> Out1/1
  errorValuesVector/1 -> Integral Error Depenent Order 2/3(errorValuesVector)
  orderValuesVector/1 -> Integral Error Depenent Order 2/4(orderValuesVector)
  setpoint/1 -> Integral Error Depenent Order 2/2(setpoint)

== system VariableOrderDifferentialEquationsToolbox/GL FVOPID - convolution type (2 inputs)/derivativeTimeDependentSubsystem ==
  time : Inport
  e : Inport  Port=2
  Action Port : ActionPort
  derivativeTimeDependentBlock : MATLAB Function  TreatAsAtomicUnit=on
  Out1 : Outport  VectorParamsAs1DForOutWhenUnconnected=off
  wires:
  time/1 -> derivativeTimeDependentBlock/1(t)
  derivativeTimeDependentBlock/1(y) -> Out1/1
  e/1 -> derivativeTimeDependentBlock/2(e)

== system VariableOrderDifferentialEquationsToolbox/GL FVOPID - convolution type (2 inputs)/integralConstantSubsystem ==
  In1 : Inport
  Action Port : ActionPort
  Out1 : Outport  VectorParamsAs1DForOutWhenUnconnected=off
  wires:
  In1/1 -> Out1/1

== system VariableOrderDifferentialEquationsToolbox/GL FVOPID - convolution type (2 inputs)/integralErrorDependentSubsystem ==
  In1 : Inport
  errorValuesVector : Inport  Port=2
  orderValuesVector : Inport  Port=3
  Action Port : ActionPort
  Integral Error Depenent Order : MATLAB Function  TreatAsAtomicUnit=on
  Out1 : Outport  VectorParamsAs1DForOutWhenUnconnected=off
  wires:
  In1/1 -> Integral Error Depenent Order/1(e)
  Integral Error Depenent Order/1(y) -> Out1/1
  errorValuesVector/1 -> Integral Error Depenent Order/2(errorValuesVector)
  orderValuesVector/1 -> Integral Error Depenent Order/3(orderValuesVector)

== system VariableOrderDifferentialEquationsToolbox/GL FVOPID - convolution type (2 inputs)/integralRatioDependentSubsystem ==
  e : Inport
  setpoint : Inport  Port=2
  errorValuesVector : Inport  Port=3
  orderValuesVector : Inport  Port=4
  Action Port : ActionPort
  Integral Error Depenent Order 2 : MATLAB Function  TreatAsAtomicUnit=on
  Out1 : Outport  VectorParamsAs1DForOutWhenUnconnected=off
  wires:
  e/1 -> Integral Error Depenent Order 2/1(e)
  Integral Error Depenent Order 2/1(y) -> Out1/1
  errorValuesVector/1 -> Integral Error Depenent Order 2/3(errorValuesVector)
  orderValuesVector/1 -> Integral Error Depenent Order 2/4(orderValuesVector)
  setpoint/1 -> Integral Error Depenent Order 2/2(setpoint)

== system VariableOrderDifferentialEquationsToolbox/GL FVOPID - convolution type (2 inputs)/integralTimeDependentSubsystem ==
  time : Inport
  e : Inport  Port=2
  Action Port : ActionPort
  integralTimeDependentBlock : MATLAB Function  TreatAsAtomicUnit=on
  Out1 : Outport  VectorParamsAs1DForOutWhenUnconnected=off
  wires:
  time/1 -> integralTimeDependentBlock/1(t)
  integralTimeDependentBlock/1(y) -> Out1/1
  e/1 -> integralTimeDependentBlock/2(e)

== matlab function VariableOrderDifferentialEquationsToolbox/GL FVOPID - Type A (2 inputs)/derivativeErrorDependentSubsystem/Derivative Error Depenent Order ==
  data: e input; y output; errorValuesVector input; orderValuesVector input
function y = derivativeOrderFunction(e, errorValuesVector, orderValuesVector)
    y = fvopidToolbox.utils.getOrderValue(e, errorValuesVector, orderValuesVector);
end

== matlab function VariableOrderDifferentialEquationsToolbox/GL FVOPID - Type A (2 inputs)/derivativeRatioDependentSubsystem/Integral Error Depenent Order 2 ==
  data: e input; setpoint input; y output; errorValuesVector input; orderValuesVector input
function y = integralOrderFunction(e, setpoint, errorValuesVector, orderValuesVector)
    y = fvopidToolbox.utils.getOrderValue(e/setpoint, errorValuesVector, orderValuesVector);
end

== matlab function VariableOrderDifferentialEquationsToolbox/GL FOPID/fopid ==
  data: e input; u output; kp input; ki input; kd input; vi input; vd input; h input; N input; saturationEnabled input; saturationLimitLow input; saturationLimitHigh input
function u = fopid(e, kp, ki, kd, vi, vd, h, N, saturationEnabled, saturationLimitLow, saturationLimitHigh)
    u = fvopidToolbox.fvopid.fopid(e, kp, ki, kd, vi, vd, h, N, saturationEnabled, saturationLimitLow, saturationLimitHigh);

== matlab function VariableOrderDifferentialEquationsToolbox/GL FVOPID - Type A (2 inputs)/derivativeTimeDependentSubsystem/derivativeTimeDependentBlock ==
  data: t input; y output; e input
function y = derivativeTimeDependentMatlabFunction(t, e)
y = 2*t + e;
end

== matlab function VariableOrderDifferentialEquationsToolbox/GL FVOPID - Type A (2 inputs)/fvopidOptimized ==
  data: e input; u output; kp input; ki input; kd input; vi input; vd input; h input; N input; saturationEnabled input; saturationLimitLow input; saturationLimitHigh input
function u = fvopidOptimized(e, kp, ki, kd, vi, vd, h, N, saturationEnabled, saturationLimitLow, saturationLimitHigh)
    u = fvopidToolbox.fvopid.fvopidTypeA(e, kp, ki, kd, vi, vd, h, N, saturationEnabled, saturationLimitLow, saturationLimitHigh);

== matlab function VariableOrderDifferentialEquationsToolbox/GL FVOPID - Type A (2 inputs)/integralErrorDependentSubsystem/Integral Error Depenent Order ==
  data: e input; y output; errorValuesVector input; orderValuesVector input
function y = integralOrderFunction(e, errorValuesVector, orderValuesVector)
    y = fvopidToolbox.utils.getOrderValue(e, errorValuesVector, orderValuesVector);
end

== matlab function VariableOrderDifferentialEquationsToolbox/GL FVOPID - Type A/derivativeErrorDependentSubsystem/Derivative Error Depenent Order ==
  data: e input; y output; errorValuesVector input; orderValuesVector input
function y = derivativeOrderFunction(e, errorValuesVector, orderValuesVector)
    y = fvopidToolbox.utils.getOrderValue(e, errorValuesVector, orderValuesVector);
end

== matlab function VariableOrderDifferentialEquationsToolbox/GL FVOPID - Type A (2 inputs)/integralRatioDependentSubsystem/Integral Error Depenent Order 2 ==
  data: e input; setpoint input; y output; errorValuesVector input; orderValuesVector input
function y = integralOrderFunction(e, setpoint, errorValuesVector, orderValuesVector)
    y = fvopidToolbox.utils.getOrderValue(e/setpoint, errorValuesVector, orderValuesVector);
end

== matlab function VariableOrderDifferentialEquationsToolbox/GL FVOPID - Type A (2 inputs)/integralTimeDependentSubsystem/integralTimeDependentBlock ==
  data: t input; y output; e input
function y = integralTimeDependentMatlabFunction(t, e)
y = 3 * t + 2 * e;
end

== matlab function VariableOrderDifferentialEquationsToolbox/GL FVOPID - convolution type (2 inputs)/derivativeErrorDependentSubsystem/Derivative Error Depenent Order ==
  data: e input; y output; errorValuesVector input; orderValuesVector input
function y = derivativeOrderFunction(e, errorValuesVector, orderValuesVector)
    y = fvopidToolbox.utils.getOrderValue(e, errorValuesVector, orderValuesVector);
end

== matlab function VariableOrderDifferentialEquationsToolbox/GL FVOPID - convolution type (2 inputs)/derivativeRatioDependentSubsystem/Integral Error Depenent Order 2 ==
  data: e input; setpoint input; y output; errorValuesVector input; orderValuesVector input
function y = integralOrderFunction(e, setpoint, errorValuesVector, orderValuesVector)
    y = fvopidToolbox.utils.getOrderValue(e/setpoint, errorValuesVector, orderValuesVector);
end

== matlab function VariableOrderDifferentialEquationsToolbox/GL FVOPID - convolution type (2 inputs)/derivativeTimeDependentSubsystem/derivativeTimeDependentBlock ==
  data: t input; y output; e input
function y = derivativeTimeDependentMatlabFunction(t, e)
y = 2*t + e;
end

== matlab function VariableOrderDifferentialEquationsToolbox/GL FVOPID - convolution type (2 inputs)/fvopidConv ==
  data: e input; u output; kp input; ki input; kd input; vi input; vd input; h input; N input; saturationEnabled input; saturationLimitLow input; saturationLimitHigh input
function u = fvopidConv(e, kp, ki, kd, vi, vd, h, N, saturationEnabled, saturationLimitLow, saturationLimitHigh)
    u = fvopidToolbox.fvopid.fvopidConv(e, kp, ki, kd, vi, vd, h, N, saturationEnabled, saturationLimitLow, saturationLimitHigh);

== matlab function VariableOrderDifferentialEquationsToolbox/GL FVOPID - convolution type (2 inputs)/integralErrorDependentSubsystem/Integral Error Depenent Order ==
  data: e input; y output; errorValuesVector input; orderValuesVector input
function y = integralOrderFunction(e, errorValuesVector, orderValuesVector)
    y = fvopidToolbox.utils.getOrderValue(e, errorValuesVector, orderValuesVector);
end

== matlab function VariableOrderDifferentialEquationsToolbox/GL FVOPID - convolution type (2 inputs)/integralRatioDependentSubsystem/Integral Error Depenent Order 2 ==
  data: e input; setpoint input; y output; errorValuesVector input; orderValuesVector input
function y = integralOrderFunction(e, setpoint, errorValuesVector, orderValuesVector)
    y = fvopidToolbox.utils.getOrderValue(e/setpoint, errorValuesVector, orderValuesVector);
end

== matlab function VariableOrderDifferentialEquationsToolbox/GL FVOPID - convolution type (2 inputs)/integralTimeDependentSubsystem/integralTimeDependentBlock ==
  data: t input; y output; e input
function y = integralTimeDependentMatlabFunction(t, e)
y = 3 * t + 2 * e;
end

== matlab function VariableOrderDifferentialEquationsToolbox/GL FVOPID - Type A/fvopidOptimized ==
  data: e input; u output; kp input; ki input; kd input; vi input; vd input; h input; N input; saturationEnabled input; saturationLimitLow input; saturationLimitHigh input
function u = fvopidOptimized(e, kp, ki, kd, vi, vd, h, N, saturationEnabled, saturationLimitLow, saturationLimitHigh)
    u = fvopidToolbox.fvopid.fvopidTypeA(e, kp, ki, kd, vi, vd, h, N, saturationEnabled, saturationLimitLow, saturationLimitHigh);

== matlab function VariableOrderDifferentialEquationsToolbox/GL FVOPID - convolution type (external orders)/fvopidConv ==
  data: e input; u output; kp input; ki input; kd input; vi input; vd input; h input; N input; saturationEnabled input; saturationLimitLow input; saturationLimitHigh input
function u = fvopidConv(e, kp, ki, kd, vi, vd, h, N, saturationEnabled, saturationLimitLow, saturationLimitHigh)
    u = fvopidToolbox.fvopid.fvopidConv(e, kp, ki, kd, vi, vd, h, N, saturationEnabled, saturationLimitLow, saturationLimitHigh);

== matlab function VariableOrderDifferentialEquationsToolbox/GL FVOPID - convolution type/derivativeErrorDependentSubsystem/Derivative Error Depenent Order ==
  data: e input; y output; errorValuesVector input; orderValuesVector input
function y = derivativeOrderFunction(e, errorValuesVector, orderValuesVector)
    y = fvopidToolbox.utils.getOrderValue(e, errorValuesVector, orderValuesVector);
end

== matlab function VariableOrderDifferentialEquationsToolbox/GL FVOPID - convolution type/derivativeRatioDependentSubsystem/Integral Error Depenent Order 2 ==
  data: e input; setpoint input; y output; errorValuesVector input; orderValuesVector input
function y = integralOrderFunction(e, setpoint, errorValuesVector, orderValuesVector)
    y = fvopidToolbox.utils.getOrderValue(e/setpoint, errorValuesVector, orderValuesVector);
end

== matlab function VariableOrderDifferentialEquationsToolbox/GL FVOPID - convolution type/derivativeTimeDependentSubsystem/derivativeTimeDependentBlock ==
  data: t input; y output; e input
function y = derivativeTimeDependentMatlabFunction(t, e)
y = 2*t + e;
end

== matlab function VariableOrderDifferentialEquationsToolbox/GL FVOPID - convolution type/fvopidConv ==
  data: e input; u output; kp input; ki input; kd input; vi input; vd input; h input; N input; saturationEnabled input; saturationLimitLow input; saturationLimitHigh input
function u = fvopidConv(e, kp, ki, kd, vi, vd, h, N, saturationEnabled, saturationLimitLow, saturationLimitHigh)
    u = fvopidToolbox.fvopid.fvopidConv(e, kp, ki, kd, vi, vd, h, N, saturationEnabled, saturationLimitLow, saturationLimitHigh);

== matlab function VariableOrderDifferentialEquationsToolbox/GL FVOPID - convolution type/integralErrorDependentSubsystem/Integral Error Depenent Order ==
  data: e input; y output; errorValuesVector input; orderValuesVector input
function y = integralOrderFunction(e, errorValuesVector, orderValuesVector)
    y = fvopidToolbox.utils.getOrderValue(e, errorValuesVector, orderValuesVector);
end

== matlab function VariableOrderDifferentialEquationsToolbox/GL FVOPID - convolution type/integralRatioDependentSubsystem/Integral Error Depenent Order 2 ==
  data: e input; setpoint input; y output; errorValuesVector input; orderValuesVector input
function y = integralOrderFunction(e, setpoint, errorValuesVector, orderValuesVector)
    y = fvopidToolbox.utils.getOrderValue(e/setpoint, errorValuesVector, orderValuesVector);
end

== matlab function VariableOrderDifferentialEquationsToolbox/GL FVOPID - convolution type/integralTimeDependentSubsystem/integralTimeDependentBlock ==
  data: t input; y output; e input
function y = integralTimeDependentMatlabFunction(t, e)
y = 3 * t + 2 * e;
end

== matlab function VariableOrderDifferentialEquationsToolbox/GL FVOPID - Type A/integralRatioDependentSubsystem/Integral Error Depenent Order 2 ==
  data: e input; setpoint input; y output; errorValuesVector input; orderValuesVector input
function y = integralOrderFunction(e, setpoint, errorValuesVector, orderValuesVector)
    y = fvopidToolbox.utils.getOrderValue(e/setpoint, errorValuesVector, orderValuesVector);
end
